simulink model "TestDiscreteTime"  (R2022a)
settings: Solver=VariableStepAuto  StartTime=0.0  StopTime=t_final  RelTol=1e-3
values from neighbouring files (symbols this model uses):
  C = eye(3)    [DAE_Circuit_main.m]
  Q = SIM.Q_0*eye(N.inputs)    [DAE_Circuit_main.m]
  R = SIM.R_0*eye(N.measur)    [DAE_Circuit_main.m]
undefined symbols (not defined in the file or in its folder): A, A_DT, B, B_DT, Iden, multiple, P_k, Ts_sample, x_0, x_0_est
settings Model: Creator=tyevans  LastModifiedBy=tyevans

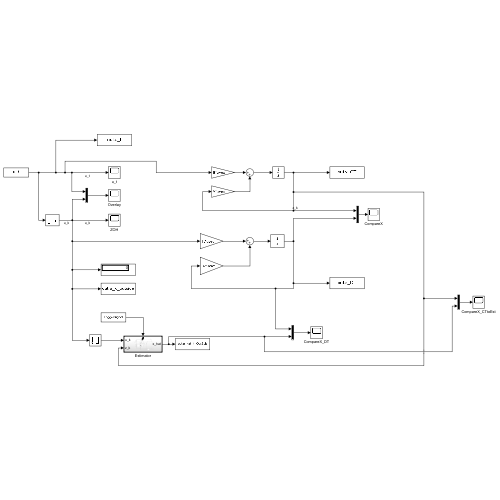
[thumbnail: Simulink's stored preview of the top-level diagram]
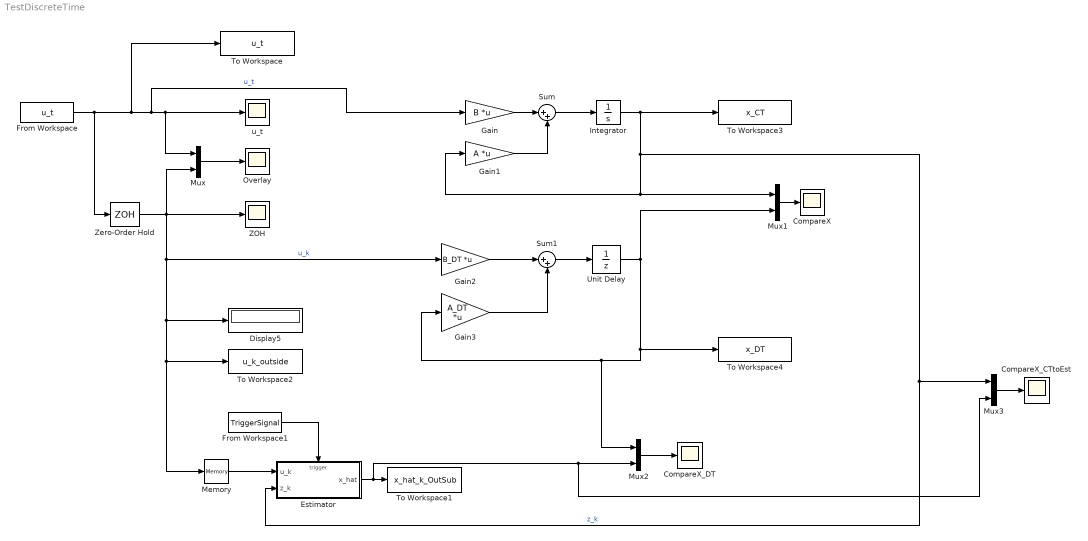
== system TestDiscreteTime ==
  CompareX : Scope
  CompareX_CTtoEst : Scope
  CompareX_DT : Scope
  Display5 : Display
  Estimator : Subsystem  TreatAsAtomicUnit=on
  From Workspace : FromWorkspace  VariableName=u_t  SampleTime=Ts_sample/multiple  OutputAfterFinalValue=Holding final value
  From Workspace1 : FromWorkspace  VariableName=TriggerSignal  Interpolate=off  OutputAfterFinalValue=Holding final value
  Gain : Gain  Gain=B  Multiplication=Matrix(K*u) (u vector)
  Gain1 : Gain  Gain=A  Multiplication=Matrix(K*u) (u vector)
  Gain2 : Gain  Gain=B_DT  Multiplication=Matrix(K*u) (u vector)
  Gain3 : Gain  Gain=A_DT  Multiplication=Matrix(K*u) (u vector)
  Integrator : Integrator  InitialCondition=x_0
  Memory : Memory
  Mux{,1..3} (4 alike) : Mux  Inputs=2
  Overlay : Scope
  Sum : Sum  Inputs=|++
  Sum1 : Sum  Inputs=|++
  To Workspace : ToWorkspace  VariableName=u_t  SaveFormat=Timeseries  SampleTime=-1
  To Workspace1 : ToWorkspace  VariableName=x_hat_k_OutSub  SampleTime=-1
  To Workspace2 : ToWorkspace  VariableName=u_k_outside  SaveFormat=Timeseries  SampleTime=-1
  To Workspace3 : ToWorkspace  VariableName=x_CT  SaveFormat=Structure With Time  SampleTime=-1
  To Workspace4 : ToWorkspace  VariableName=x_DT  SaveFormat=Timeseries  SampleTime=-1
  Unit Delay : UnitDelay  InitialCondition=x_0  SampleTime=-1  HasFrameUpgradeWarning=on
  ZOH : Scope
  Zero-Order Hold : ZeroOrderHold  SampleTime=Ts_sample
  u_t : Scope
  wires:
  From Workspace/1 -> Zero-Order Hold/1, To Workspace/1, u_t/1, Mux/1, Gain/1  "u_t"
  Mux/1 -> Overlay/1
  Gain/1 -> Sum/1
  Gain1/1 -> Sum/2
  Sum/1 -> Integrator/1
  Gain3/1 -> Sum1/2
  Unit Delay/1 -> Mux2/1, Gain3/1, To Workspace4/1, Mux1/2
  Sum1/1 -> Unit Delay/1
  Gain2/1 -> Sum1/1
  Mux1/1 -> CompareX/1
  Zero-Order Hold/1 -> Memory/1, To Workspace2/1, Display5/1, Gain2/1, Mux/2, ZOH/1  "u_k"
  Integrator/1 -> To Workspace3/1, Mux1/1, Gain1/1, Mux3/1, Estimator/2(z_k)  "z_k"
  Estimator/1(x_hat) -> Mux3/2, Mux2/2, To Workspace1/1
  From Workspace1/1 -> Estimator/Trigger
  Mux2/1 -> CompareX_DT/1
  Mux3/1 -> CompareX_CTtoEst/1
  Memory/1 -> Estimator/1(u_k)

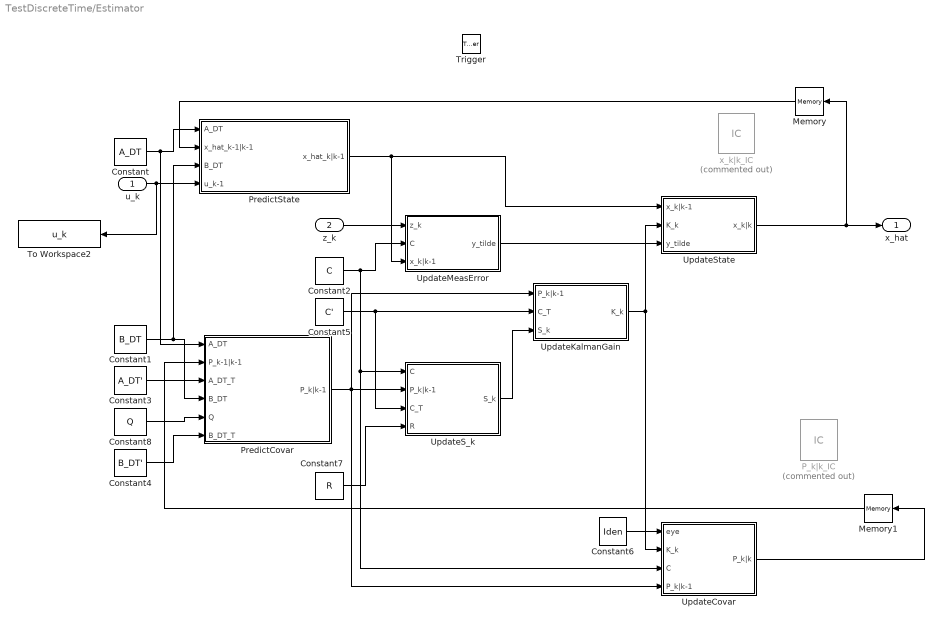
== system TestDiscreteTime/Estimator ==
  u_k : Inport
  z_k : Inport  Port=2
  Trigger : TriggerPort  VariantControl=(inherit)
  Constant : Constant  Value=A_DT  VectorParams1D=off
  Constant1 : Constant  Value=B_DT  VectorParams1D=off
  Constant2 : Constant  Value=C  VectorParams1D=off
  Constant3 : Constant  Value=A_DT'  VectorParams1D=off
  Constant4 : Constant  Value=B_DT'  VectorParams1D=off
  Constant5 : Constant  Value=C'  VectorParams1D=off
  Constant6 : Constant  Value=Iden  VectorParams1D=off
  Constant7 : Constant  Value=R  VectorParams1D=off
  Constant8 : Constant  Value=Q  VectorParams1D=off
  Memory : Memory  InitialCondition=x_0_est  InheritSampleTime=on
  Memory1 : Memory  InitialCondition=P_k(:,:,1)  InheritSampleTime=on
  P_k|k_IC : InitialCondition  Commented=on  Value=P_k(:,:,1)
  PredictCovar : Subsystem
  PredictState : Subsystem
  To Workspace2 : ToWorkspace  VariableName=u_k  SaveFormat=Timeseries  SampleTime=-1
  UpdateCovar : Subsystem
  UpdateKalmanGain : Subsystem
  UpdateMeasError : Subsystem
  UpdateS_k : Subsystem
  UpdateState : Subsystem
  x_k|k_IC : InitialCondition  Commented=on  Value=x_0_est
  x_hat : Outport
  wires:
  UpdateS_k/1(S_k) -> UpdateKalmanGain/3(S_k)
  Constant6/1 -> UpdateCovar/1(eye)
  Constant3/1 -> PredictCovar/3(A_DT_T)
  UpdateMeasError/1(y_tilde) -> UpdateState/3(y_tilde)
  Constant7/1 -> UpdateS_k/4(R)
  Constant4/1 -> PredictCovar/6(B_DT_T)
  Constant8/1 -> PredictCovar/5(Q)
  z_k/1 -> UpdateMeasError/1(z_k)
  u_k/1 -> To Workspace2/1, PredictState/4(u_k-1)
  UpdateKalmanGain/1(K_k) -> UpdateState/2(K_k), UpdateCovar/2(K_k)
  PredictState/1(x_hat_k|k-1) -> UpdateMeasError/3(x_k|k-1), UpdateState/1(x_k|k-1)
  PredictCovar/1(P_k|k-1) -> UpdateS_k/2(P_k|k-1), UpdateCovar/4(P_k|k-1), UpdateKalmanGain/1(P_k|k-1)
  Constant5/1 -> UpdateS_k/3(C_T), UpdateKalmanGain/2(C_T)
  Constant2/1 -> UpdateS_k/1(C), UpdateCovar/3(C), UpdateMeasError/2(C)
  Constant1/1 -> PredictState/3(B_DT), PredictCovar/4(B_DT)
  Constant/1 -> PredictState/1(A_DT), PredictCovar/1(A_DT)
  Memory/1 -> PredictState/2(x_hat_k-1|k-1)
  UpdateState/1(x_k|k) -> Memory/1, x_hat/1
  UpdateCovar/1(P_k|k) -> Memory1/1
  Memory1/1 -> PredictCovar/2(P_k-1|k-1)

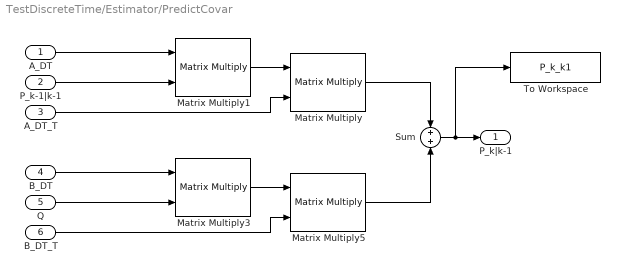
== system TestDiscreteTime/Estimator/PredictCovar ==
  A_DT : Inport
  P_k-1|k-1 : Inport  Port=2
  A_DT_T : Inport  Port=3
  B_DT : Inport  Port=4
  Q : Inport  Port=5
  B_DT_T : Inport  Port=6
  Matrix Multiply{,1,3,5} (4 alike) : Product  Multiplication=Matrix(*)
  Sum : Sum
  To Workspace : ToWorkspace  VariableName=P_k_k1  SampleTime=-1
  P_k|k-1 : Outport
  wires:
  Sum/1 -> To Workspace/1, P_k|k-1/1
  A_DT/1 -> Matrix Multiply1/1
  P_k-1|k-1/1 -> Matrix Multiply1/2
  A_DT_T/1 -> Matrix Multiply/2
  Matrix Multiply1/1 -> Matrix Multiply/1
  B_DT/1 -> Matrix Multiply3/1
  Q/1 -> Matrix Multiply3/2
  B_DT_T/1 -> Matrix Multiply5/2
  Matrix Multiply3/1 -> Matrix Multiply5/1
  Matrix Multiply/1 -> Sum/1
  Matrix Multiply5/1 -> Sum/2

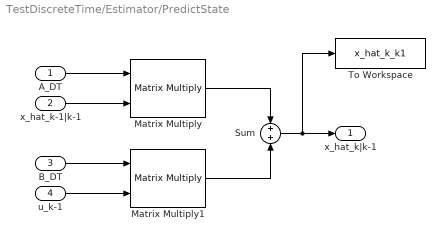
== system TestDiscreteTime/Estimator/PredictState ==
  A_DT : Inport
  x_hat_k-1|k-1 : Inport  Port=2
  B_DT : Inport  Port=3
  u_k-1 : Inport  Port=4
  Matrix Multiply : Product  Multiplication=Matrix(*)
  Matrix Multiply1 : Product  Multiplication=Matrix(*)
  Sum : Sum
  To Workspace : ToWorkspace  VariableName=x_hat_k_k1  SampleTime=-1
  x_hat_k|k-1 : Outport
  wires:
  A_DT/1 -> Matrix Multiply/1
  x_hat_k-1|k-1/1 -> Matrix Multiply/2
  B_DT/1 -> Matrix Multiply1/1
  u_k-1/1 -> Matrix Multiply1/2
  Matrix Multiply/1 -> Sum/1
  Matrix Multiply1/1 -> Sum/2
  Sum/1 -> To Workspace/1, x_hat_k|k-1/1

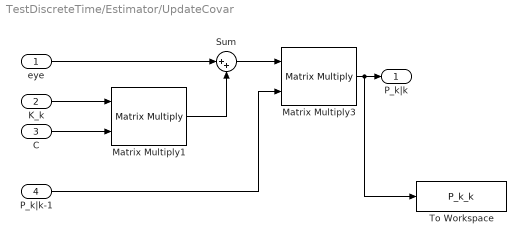
== system TestDiscreteTime/Estimator/UpdateCovar ==
  eye : Inport
  K_k : Inport  Port=2
  C : Inport  Port=3
  P_k|k-1 : Inport  Port=4
  Matrix Multiply1 : Product  Multiplication=Matrix(*)
  Matrix Multiply3 : Product  Multiplication=Matrix(*)
  Sum : Sum  Inputs=|++
  To Workspace : ToWorkspace  VariableName=P_k_k  SampleTime=-1
  P_k|k : Outport
  wires:
  K_k/1 -> Matrix Multiply1/1
  C/1 -> Matrix Multiply1/2
  Matrix Multiply3/1 -> To Workspace/1, P_k|k/1
  P_k|k-1/1 -> Matrix Multiply3/2
  eye/1 -> Sum/1
  Matrix Multiply1/1 -> Sum/2
  Sum/1 -> Matrix Multiply3/1

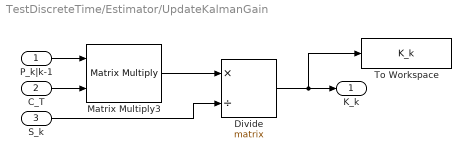
== system TestDiscreteTime/Estimator/UpdateKalmanGain ==
  P_k|k-1 : Inport
  C_T : Inport  Port=2
  S_k : Inport  Port=3
  Divide : Product  Inputs=*/  Multiplication=Matrix(*)
  Matrix Multiply3 : Product  Multiplication=Matrix(*)
  To Workspace : ToWorkspace  VariableName=K_k  SampleTime=-1
  K_k : Outport
  wires:
  Matrix Multiply3/1 -> Divide/1
  Divide/1 -> To Workspace/1, K_k/1
  P_k|k-1/1 -> Matrix Multiply3/1
  C_T/1 -> Matrix Multiply3/2
  S_k/1 -> Divide/2

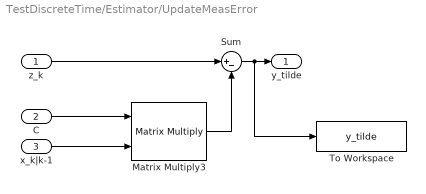
== system TestDiscreteTime/Estimator/UpdateMeasError ==
  z_k : Inport
  C : Inport  Port=2
  x_k|k-1 : Inport  Port=3
  Matrix Multiply3 : Product  Multiplication=Matrix(*)
  Sum : Sum  Inputs=|+-
  To Workspace : ToWorkspace  VariableName=y_tilde  SampleTime=-1
  y_tilde : Outport
  wires:
  Matrix Multiply3/1 -> Sum/2
  Sum/1 -> To Workspace/1, y_tilde/1
  z_k/1 -> Sum/1
  x_k|k-1/1 -> Matrix Multiply3/2
  C/1 -> Matrix Multiply3/1

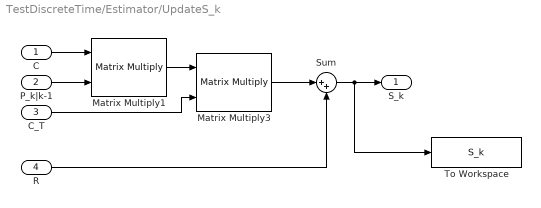
== system TestDiscreteTime/Estimator/UpdateS_k ==
  C : Inport
  P_k|k-1 : Inport  Port=2
  C_T : Inport  Port=3
  R : Inport  Port=4
  Matrix Multiply1 : Product  Multiplication=Matrix(*)
  Matrix Multiply3 : Product  Multiplication=Matrix(*)
  Sum : Sum  Inputs=|++
  To Workspace : ToWorkspace  VariableName=S_k  SampleTime=-1
  S_k : Outport
  wires:
  Matrix Multiply1/1 -> Matrix Multiply3/1
  Matrix Multiply3/1 -> Sum/1
  Sum/1 -> To Workspace/1, S_k/1
  C/1 -> Matrix Multiply1/1
  P_k|k-1/1 -> Matrix Multiply1/2
  C_T/1 -> Matrix Multiply3/2
  R/1 -> Sum/2

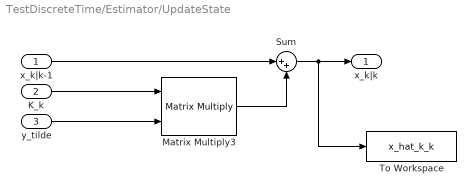
== system TestDiscreteTime/Estimator/UpdateState ==
  x_k|k-1 : Inport
  K_k : Inport  Port=2
  y_tilde : Inport  Port=3
  Matrix Multiply3 : Product  Multiplication=Matrix(*)
  Sum : Sum  Inputs=|++
  To Workspace : ToWorkspace  VariableName=x_hat_k_k  SaveFormat=Structure With Time  SampleTime=-1
  x_k|k : Outport
  wires:
  K_k/1 -> Matrix Multiply3/1
  y_tilde/1 -> Matrix Multiply3/2
  x_k|k-1/1 -> Sum/1
  Matrix Multiply3/1 -> Sum/2
  Sum/1 -> To Workspace/1, x_k|k/1
